simulink model "Cularis_openloop"  (Simulink 8.6)
settings: Solver=FixedStepAuto  SolverMode=SingleTasking  StartTime=0.0  StopTime=uavsim.simConfig.tsim  FixedStep=uavsim.simConfig.tsample_model  RelTol=1
model workspace (MAT data in the model file):
  VortexSig = Simulink.Signal
  VortexSig.DataType = 'Bus: VortexStates'
  VortexSig.Units = 'auto'
  VortexSig.Dimensions = [10 1]
  VortexSig.DimensionsMode = 'Fixed'
  VortexSig.Complexity = 'real'
  VortexSig.SampleTime = -1
  VortexSig.SamplingMode = 'auto'
  VortexSig.InitialValue = 'VortexStates_MATLABStruct_array'
undefined symbols (not defined in the file): uavsim
libraries: aerolibanimutils x1, uavsimBlockset_Cularis_withUAV3D x1
settings Model: Creator=mstolle  LastModifiedBy=j.bolting  ExtModeTrigDuration=100
settings SolverCC: ZcThreshold=1e-5  ZeroCrossAlgorithm=Adaptive  AlgebraicLoopSolver=LineSearch  AutoInsertRateTranBlk=on
settings DataIOCC: LimitDataPoints=off  SaveFinalState=on  SaveFormat=StructureWithTime  SignalLoggingSaveFormat=Dataset  SaveOutput=off  SaveState=on  DSMLogging=off  InspectSignalLogs=on  StateSaveName=tmp_raccel_xout
settings OptimizationCC: BlockReduction=off  OptimizeBlockIOStorage=off  BufferReuse=off  GlobalBufferReuse=off  ExpressionFolding=off  LocalBlockOutputs=off  EfficientMapNaN2IntZero=off  SimCompilerOptimization=on
settings DebuggingCC: UnderspecifiedInitializationDetection=Simplified  MergeDetectMultiDrivingBlocksExec=error  IgnoredZcDiagnostic=none  FcnCallInpInsideContextMsg=EnableAllAsError  BusObjectLabelMismatch=error
settings HardwareCC: TargetBitPerPointer=64  TargetLongLongMode=on  TargetIntDivRoundTo=Zero  TargetEndianess=LittleEndian  TargetWordSize=64  TargetHWDeviceType=MATLAB Host  ProdEqTarget=off
settings ModelReferenceCC: UpdateModelReferenceTargets=IfOutOfDate  ModelReferenceNumInstancesAllowed=Single  ModelReferenceMinAlgLoopOccurrences=on
settings SFSimCC: SFSimEcho=off
settings RTWCC: SystemTargetFile=raccel.tlc  TemplateMakefile=raccel_default_tmf  RTWVerbose=off  RTWUseSimCustomCode=on
settings CodeAppCC: GenerateComments=off  MaxIdLength=128  SimulinkBlockComments=off
settings RaccelTargetCC: ERTMultiwordTypeDef=System defined  ERTMultiwordLength=256  GeneratePreprocessorConditionals=Use local settings  ERTFirstTimeCompliant=off  MultiInstanceERTCode=off  ENABLE_SLEXEC_SSBRIDGE=0  RTWCAPIParams=on
settings ConfigComp: CovSFcnEnable=off
settings ConfigurationSet: Description=SimMechanics 2G

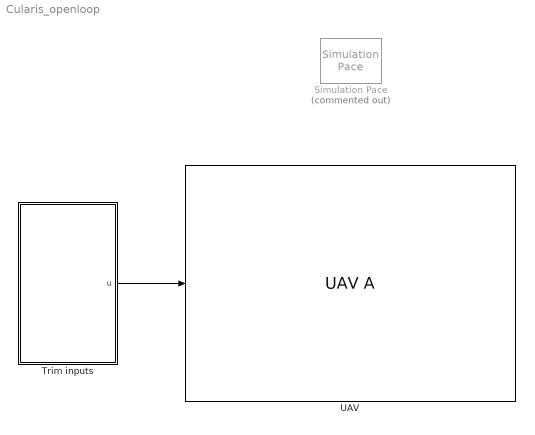
== system Cularis_openloop ==
  Simulation Pace : aerolibanimutils/Simulation Pace  Commented=on  SimulationPace=1  SleepMode=MATLAB Thread  OutputPaceError=off  SampleTime=-1
  Trim inputs : Subsystem  SystemSampleTime=uavsim.ap.hardware.dt_attitudeloops_s
  UAV : uavsimBlockset_Cularis_withUAV3D/UAV A  aircraftmask_phithetapsi0=uavsim.formation(1).phithetapsi0  aircraftmask_p0_NED_m=uavsim.formation(1).p0_NED'  aircraftmask_originNED_ECEF_rrm=uavsim.originNED_ECEF_radradm  aircraftmask_pqr0=uavsim.formation(1).omega0  aircraftmask_uvw0=uavsim.formation(1).uvw0  aircraftmask_phithetapsi_trim=uavsim.formation(1).phithetapsi0  aircraftmask_ID=1  aircraftmask_wakevortexenabled=off  aircraftmask_navigationLaw=-1  uavsim=uavsim  leaderID=0  aircraftmask_displayUAV3D=on  aircraftmask_displayVortices=off
  wires:
  Trim inputs/1(u) -> UAV/1

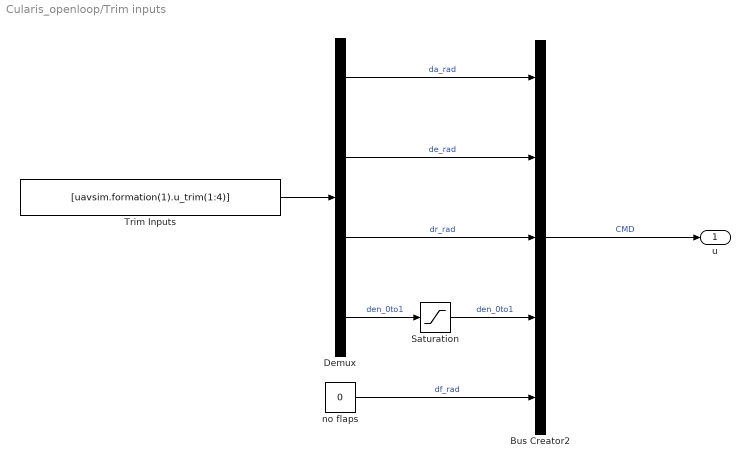
== system Cularis_openloop/Trim inputs ==
  Bus Creator2 : BusCreator  Inputs=5  OutDataTypeStr=Bus: CMD  NonVirtualBus=on
  Demux : Demux
  Saturation : Saturate  UpperLimit=1  LowerLimit=0
  Trim Inputs : Constant  Value=[uavsim.formation(1).u_trim(1:4)]
  no flaps : Constant  Value=0
  u : Outport  OutDataTypeStr=Bus: CMD
  wires:
  no flaps/1 -> Bus Creator2/5  "df_rad"
  Trim Inputs/1 -> Demux/1
  Demux/2 -> Bus Creator2/2  "de_rad"
  Demux/1 -> Bus Creator2/1  "da_rad"
  Saturation/1 -> Bus Creator2/4  "den_0to1"
  Demux/3 -> Bus Creator2/3  "dr_rad"
  Bus Creator2/1 -> u/1  "CMD"
  Demux/4 -> Saturation/1  "den_0to1"
